simulink model "sequential"  (Simulink 7.7)
settings: Solver=FixedStepDiscrete  StartTime=0.0  StopTime=inf  RelTol=1e-3
undefined symbols (not defined in the file): darwinop_communication_setup
libraries: simulink x10, lib_darwinop x1
settings Model: Creator=eleve  LastModifiedBy=eleve  BufferReuse=off
settings DataIOCC: SignalLoggingSaveFormat=Dataset
settings OptimizationCC: BlockReduction=off  BufferReuse=off  ExpressionDepthLimit=128  OptimizeModelRefInitCode=on  LifeSpan=Inf
settings DebuggingCC: AlgebraicLoopMsg=none  SolverPrmCheckMsg=none  FcnCallInpInsideContextMsg=Enable All  UnconnectedInputMsg=none  UnconnectedOutputMsg=none  UnconnectedLineMsg=none
settings HardwareCC: ProdEndianess=LittleEndian  ProdHWDeviceType=Generic->32-bit Embedded Processor
settings RTWCC: SystemTargetFile=darwinoplib.tlc  GenCodeOnly=on  TemplateMakefile=darwinoplib.tmf  Description=DarwinOP code generator  ProcessScript=darwinoplib_make_rtw_hook  TargetLang=C++
settings CodeAppCC: IgnoreCustomStorageClasses=off  CustomSymbolStrType=$N$R$M_T
settings STFCustomTargetCC: CombineOutputUpdateFcns=on  ERTCustomFileBanners=on  SupportContinuousTime=off  SupportNonInlinedSFcns=off  SystemTargetFile=darwinoplib.tlc
settings ERTTargetCC: MultiwordLength=2048  ParMdlRefBuildCompliant=off  CompOptLevelCompliant=off  ERTFirstTimeCompliant=off  ModelStepFunctionPrototypeControlCompliant=off  CPPClassGenCompliant=off  InlinedParameterPlacement=NonHierarchical  ERTCustomFileTemplate=darwinoplib_main.tlc  ConvertIfToSwitch=off  SuppressUnreachableDefaultCases=off
settings CustomProperty: DataType=string  Value=192.168.123.1

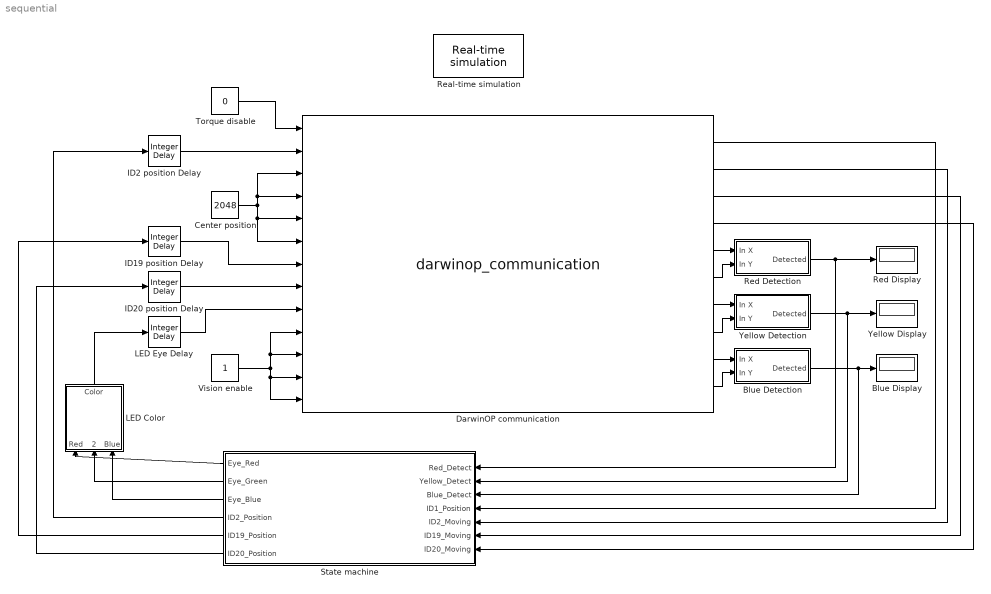
== system sequential ==
  Blue Detection : Subsystem
  Blue Display : Display
  Center position : Constant  Value=2048
  DarwinOP communication : M-S-Function  StartFcn=darwinop_communication_setup('StartFcn');  StopFcn=darwinop_communication_setup('StopFcn');  FunctionName=darwinop_communication  Parameters=IP,Port,Protocol,SampleTime,Frame,ReadIndex,WriteIndex  mask{IP=192.168.123.1, Port=1234, Protocol=tcp, SampleTime=0.05, Frame=[ 2 1 36 2 3 1 24 1 0 2 2 46 1 3 2 30 2 0 0 3 3 30 2 0 0 3 4 30 2 0 0 3 5 30 2 0 0 3 6 30 2 0 0 2 19 46 1 3 19 30 2 0 0 2 20 46 1 3 20 30 2 0 0 3 200 28 2 0 0 17 1 50 4 17 1 70 4 17 1 90 4 18 1 1 1 0 18 1 3 3 0 0 0], ReadIndex=[ 1 2;3 1;4 1;5 1;6 2;8 2;10 2;12 2;14 2;16 2], WriteIndex=[ 9 1;18 2;24 2;30 2;36 2;42 2;52 2;62 2;68 2;86 1;91 1;92 1;93 1]}
      settings: DeleteFcn=darwinop_communication_setup('DeleteFcn');  ModelCloseFcn=darwinop_communication_setup('ModelCloseFcn');  NameChangeFcn=darwinop_communication_setup('NameChangeFcn');  OpenFcn=darwinop_communication_setup('OpenFcn');
      mask StyleString: edit,edit,popup(tcp|udp),edit,edit,edit,edit
      mask Display:
      | image(imread('darwin-blk.jpg'))
      | 
      | port_label('output',1,'Right Shoulder Pitch(1)/Position')
      | port_label('output',2,'Left Shoulder Pitch(2)/Moving')
      | port_label('output',3,'Head Pan(19)/Moving')
      | port_label('output',4,'Head Tilt(20)/Moving')
      | port_label('output',5,'Vision(1)/Red X')
      | port_label('output',6,'Vision(1)/Red Y')
      | port_label('output',7,'Vision(1)/Yellow X')
      | port_label('output',8,'Vision(1)/Yellow Y')
      | port_label('output',9,'Vision(1)/Blue X')
      | port_label('output',10,'Vision(1)/Blue Y')
      | 
      | port_label('input',1,'Right Shoulder Pitch(1)/Torque Enable')
      | port_label('input',2,'Left Shoulder Pitch(2)/Goal Position')
      | port_label('input',3,'Right Shoulder Roll(3)/Goal Position')
      | port_label('input',4,'Left Shoulder Roll(4)/Goal Position')
      | port_label('input',5,'Right Elbow(5)/Goal Position')
      | port_label('input',6,'Left Elbow(6)/Goal Position')
      | port_label('input',7,'Head Pan(19)/Goal Position')
      | port_label('input',8,'Head Tilt(20)/Goal Position')
      | port_label('input',9,'Sub controller(200)/LED Eye')
      | port_label('input',10,'Vision(1)/Enable')
      | port_label('input',11,'Vision(1)/Red Enable')
      | port_label('input',12,'Vision(1)/Yellow enable')
      | port_label('input',13,'Vision(1)/Blue enable')
  ID19 position Delay : simulink/Discrete/Integer Delay  NumDelays=1  vinit=2048  samptime=-1
  ID2 position Delay : simulink/Discrete/Integer Delay  NumDelays=1  vinit=2048  samptime=-1
  ID20 position Delay : simulink/Discrete/Integer Delay  NumDelays=1  vinit=2048  samptime=-1
  LED Color : Subsystem
  LED Eye Delay : simulink/Discrete/Integer Delay  NumDelays=1  vinit=2048  samptime=-1
  Real-time simulation : lib_darwinop/Real-time simulation  TimeScalingFactor=1
  Red Detection : Subsystem
  Red Display : Display
  State machine : Stateflow chart  TreatAsAtomicUnit=on
      settings: PermitHierarchicalResolution=ParametersOnly
  Torque disable : Constant  Value=0
  Vision enable : Constant
  Yellow Detection : Subsystem
  Yellow Display : Display
  wires:
  Red Detection/1(Detected) -> State machine/1(Red_Detect), Red Display/1
  Yellow Detection/1(Detected) -> State machine/2(Yellow_Detect), Yellow Display/1
  Blue Detection/1(Detected) -> State machine/3(Blue_Detect), Blue Display/1
  LED Color/1(Color) -> LED Eye Delay/1
  Vision enable/1 -> DarwinOP communication/12, DarwinOP communication/13, DarwinOP communication/11, DarwinOP communication/10
  Torque disable/1 -> DarwinOP communication/1
  Center position/1 -> DarwinOP communication/4, DarwinOP communication/3, DarwinOP communication/5, DarwinOP communication/6
  ID2 position Delay/1 -> DarwinOP communication/2
  ID19 position Delay/1 -> DarwinOP communication/7
  State machine/1(Eye_Red) -> LED Color/1(Red)
  State machine/2(Eye_Green) -> LED Color/2(Green)
  State machine/3(Eye_Blue) -> LED Color/3(Blue)
  State machine/4(ID2_Position) -> ID2 position Delay/1
  State machine/5(ID19_Position) -> ID19 position Delay/1
  DarwinOP communication/1 -> State machine/4(ID1_Position)
  DarwinOP communication/2 -> State machine/5(ID2_Moving)
  DarwinOP communication/3 -> State machine/6(ID19_Moving)
  DarwinOP communication/10 -> Blue Detection/2(In Y)
  DarwinOP communication/9 -> Blue Detection/1(In X)
  DarwinOP communication/8 -> Yellow Detection/2(In Y)
  DarwinOP communication/7 -> Yellow Detection/1(In X)
  DarwinOP communication/6 -> Red Detection/2(In Y)
  DarwinOP communication/5 -> Red Detection/1(In X)
  ID20 position Delay/1 -> DarwinOP communication/8
  State machine/6(ID20_Position) -> ID20 position Delay/1
  DarwinOP communication/4 -> State machine/7(ID20_Moving)
  LED Eye Delay/1 -> DarwinOP communication/9

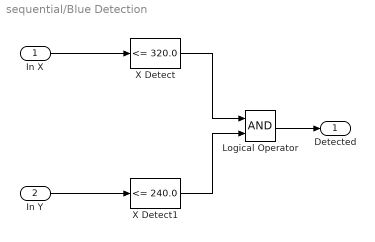
== system sequential/Blue Detection ==
  In X : Inport
  In Y : Inport  Port=2
  Logical Operator : Logic  AllPortsSameDT=off  OutDataTypeStr=boolean
  X Detect : simulink/Logic and Bit Operations/Compare To Constant  relop=<=  const=320.0  LogicOutDataTypeMode=boolean
  X Detect1 : simulink/Logic and Bit Operations/Compare To Constant  relop=<=  const=240.0  LogicOutDataTypeMode=boolean
  Detected : Outport
  wires:
  Logical Operator/1 -> Detected/1
  X Detect/1 -> Logical Operator/1
  X Detect1/1 -> Logical Operator/2
  In Y/1 -> X Detect1/1
  In X/1 -> X Detect/1

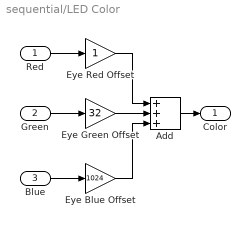
== system sequential/LED Color ==
  Red : Inport
  Green : Inport  Port=2
  Blue : Inport  Port=3
  Add : Sum  Inputs=+++
  Eye Blue Offset : Gain  Gain=1024
  Eye Green Offset : Gain  Gain=32
  Eye Red Offset : Gain
  Color : Outport
  wires:
  Red/1 -> Eye Red Offset/1
  Eye Green Offset/1 -> Add/2
  Eye Blue Offset/1 -> Add/3
  Green/1 -> Eye Green Offset/1
  Blue/1 -> Eye Blue Offset/1
  Eye Red Offset/1 -> Add/1
  Add/1 -> Color/1

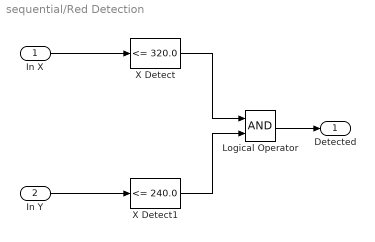
== system sequential/Red Detection ==
  In X : Inport
  In Y : Inport  Port=2
  Logical Operator : Logic  AllPortsSameDT=off  OutDataTypeStr=boolean
  X Detect : simulink/Logic and Bit Operations/Compare To Constant  relop=<=  const=320.0  LogicOutDataTypeMode=boolean
  X Detect1 : simulink/Logic and Bit Operations/Compare To Constant  relop=<=  const=240.0  LogicOutDataTypeMode=boolean
  Detected : Outport
  wires:
  Logical Operator/1 -> Detected/1
  X Detect/1 -> Logical Operator/1
  X Detect1/1 -> Logical Operator/2
  In Y/1 -> X Detect1/1
  In X/1 -> X Detect/1

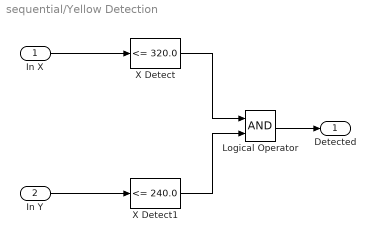
== system sequential/Yellow Detection ==
  In X : Inport
  In Y : Inport  Port=2
  Logical Operator : Logic  AllPortsSameDT=off  OutDataTypeStr=boolean
  X Detect : simulink/Logic and Bit Operations/Compare To Constant  relop=<=  const=320.0  LogicOutDataTypeMode=boolean
  X Detect1 : simulink/Logic and Bit Operations/Compare To Constant  relop=<=  const=240.0  LogicOutDataTypeMode=boolean
  Detected : Outport
  wires:
  Logical Operator/1 -> Detected/1
  X Detect/1 -> Logical Operator/1
  X Detect1/1 -> Logical Operator/2
  In Y/1 -> X Detect1/1
  In X/1 -> X Detect/1

== stateflow chart State machine ==
  state Initialisation
    entry: Eye_Red = 0;
    entry: Eye_Green = 0;
    entry: Eye_Blue = 0;
    entry: ID2_Position = 2048;
    entry: ID19_Position = 2048;
    entry: ID20_Position = 2048;
  state Yes_Up
    entry: ID20_Position = 2248;
    entry: Eye_Green = 31;
    entry: Eye_Red = 31;
  state No_Left
    entry: ID19_Position = 2248;
    entry: Eye_Red = 31;
  state Yes_Down_Wait
  state Yes_Up_Wait
  state No_Left_Wait
  state No_Right_Wait
  state Yes_Down
    entry: ID20_Position = 1848;
  state Copy
    entry: Eye_Blue = 31;
    during: ID2_Position = 4095 - ID1_Position;
  state No_Right
    entry: ID19_Position = 1848;
  (default) -> Initialisation
  No_Left -> Initialisation [order 2] : [Red_Detect == 0]
  Initialisation -> Yes_Up [order 2] : [Red_Detect == 0 && Yellow_Detect == 1 && Blue_Detect == 0]
  Yes_Up -> Initialisation [order 2] : [Yellow_Detect == 0]
  Initialisation -> No_Left [order 1] : [Red_Detect == 1 && Yellow_Detect == 0 && Blue_Detect == 0]
  Yes_Down_Wait -> Yes_Up : [ID20_Moving == 0]
  Yes_Up -> Yes_Up_Wait [order 1] : [ID20_Moving == 1 && Yellow_Detect == 1]
  Copy -> Initialisation : [Blue_Detect == 0]
  Initialisation -> Copy [order 3] : [Red_Detect == 0 && Yellow_Detect == 0 && Blue_Detect == 1]
  No_Left -> No_Left_Wait [order 1] : [ID19_Moving == 1 && Red_Detect == 1]
  No_Right_Wait -> No_Left : [ID19_Moving == 0]
  Yes_Up_Wait -> Yes_Down : [ID20_Moving == 0]
  Yes_Down -> Yes_Down_Wait : [ID20_Moving == 1]
  No_Left_Wait -> No_Right : [ID19_Moving == 0]
  No_Right -> No_Right_Wait : [ID19_Moving == 1]
  data: Red_Detect input boolean; Yellow_Detect input boolean; Blue_Detect input boolean; ID1_Position input double; ID2_Moving input double; ID19_Moving input double; Eye_Red output double; Eye_Green output double; Eye_Blue output double; ID2_Position output double; ID19_Position output double; ID20_Moving input double; ID20_Position output double
